simulink model "modelo_robot_6dof_dindir"  (R2023b)
settings: Solver=ode45  StartTime=0.0  StopTime=tsim  MaxStep=1e-2
undefined symbols (not defined in the file): robot_params, tau_L, tau_Rref
settings Model: Creator=HP  LastModifiedBy=HP

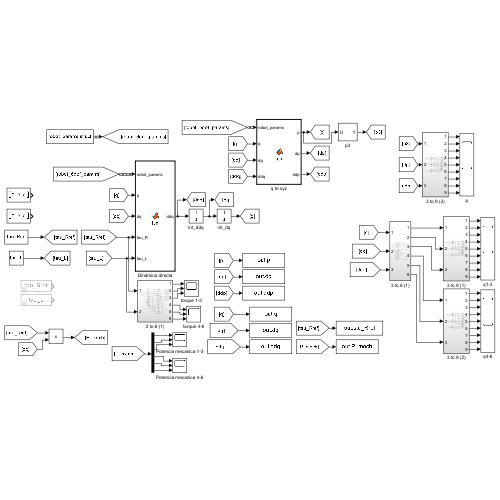
[thumbnail: Simulink's stored preview of the top-level diagram]
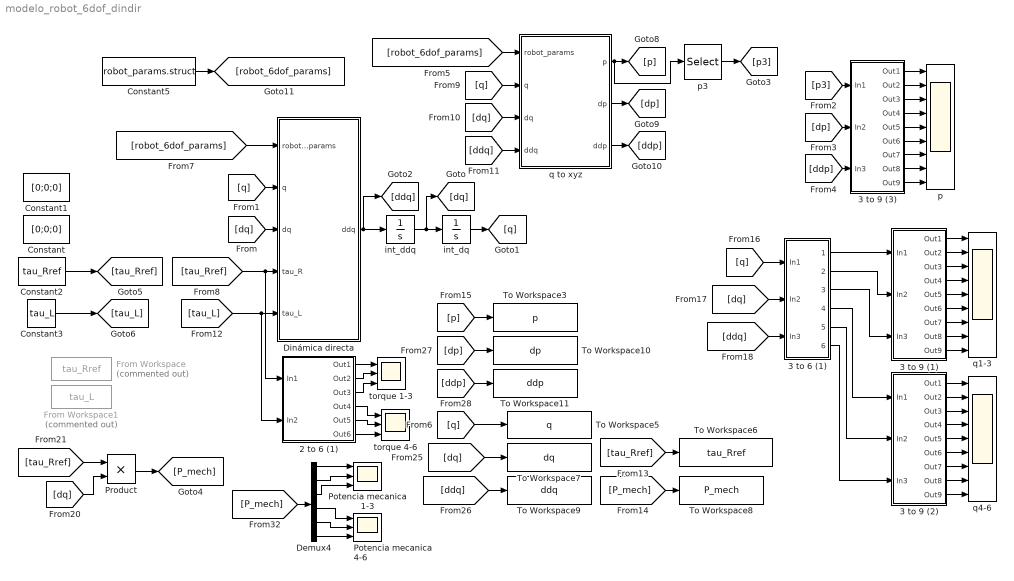
== system modelo_robot_6dof_dindir ==
  2 to 6 (1) : Subsystem
  3 to 6 (1) : Subsystem
  3 to 9 (1) : Subsystem
  3 to 9 (2) : Subsystem
  3 to 9 (3) : Subsystem
  Constant : Constant  Value=[0;0;0]
  Constant1 : Constant  Value=[0;0;0]
  Constant2 : Constant  Value=tau_Rref
  Constant3 : Constant  Value=tau_L
  Constant5 : Constant  Value=robot_params.struct  OutDataTypeStr=Bus: robot_params_bus
  Demux4 : Demux  Outputs=6
  Dinámica directa : MATLAB Function  TreatAsAtomicUnit=on
  From Workspace : FromWorkspace  Commented=on  VariableName=tau_Rref
  From Workspace1 : FromWorkspace  Commented=on  VariableName=tau_L
  Potencia mecanica 1-3 : Scope  NumInputPorts=3
  Potencia mecanica 4-6 : Scope  NumInputPorts=3
  Product : Product
  To Workspace10 : ToWorkspace  VariableName=dp  SaveFormat=Timeseries  SampleTime=-1
  To Workspace11 : ToWorkspace  VariableName=ddp  SaveFormat=Timeseries  SampleTime=-1
  To Workspace3 : ToWorkspace  VariableName=p  SaveFormat=Timeseries  SampleTime=-1
  To Workspace5 : ToWorkspace  VariableName=q  SaveFormat=Timeseries  SampleTime=-1
  To Workspace6 : ToWorkspace  VariableName=tau_Rref  SaveFormat=Timeseries  SampleTime=-1
  To Workspace7 : ToWorkspace  VariableName=dq  SaveFormat=Timeseries  SampleTime=-1
  To Workspace8 : ToWorkspace  VariableName=P_mech  SaveFormat=Timeseries  SampleTime=-1
  To Workspace9 : ToWorkspace  VariableName=ddq  SaveFormat=Timeseries  SampleTime=-1
  int_ddq : Integrator  InitialCondition=[0;0;0;0;0;0]
  int_dq : Integrator  InitialCondition=[0;-1.3744;0;1.669;0;0]
  p : Scope  NumInputPorts=9
  p3 : Selector  NumberOfDimensions=2  InputPortWidth=3  IndexOptions=Index vector (dialog),Index vector (dialog)  Indices=[1:3],3  OutputSizes=1,1
  q to xyz : MATLAB Function  TreatAsAtomicUnit=on
  q1-3 : Scope  NumInputPorts=9
  q4-6 : Scope  NumInputPorts=9
  torque 1-3 : Scope  NumInputPorts=3
  torque 4-6 : Scope  NumInputPorts=3
  wires:
  Dinámica directa/1(ddq) -> [ddq], int_ddq/1
  int_ddq/1 -> [dq], int_dq/1
  int_dq/1 -> [q]
  [dq] -> Dinámica directa/3(dq)
  [q] -> Dinámica directa/2(q)
  [tau_L] -> 2 to 6 (1)/2(In2), Dinámica directa/5(tau_L)
  Constant5/1 -> [robot_6dof_params]
  [robot_6dof_params] -> Dinámica directa/1(robot_params)
  [tau_Rref] -> 2 to 6 (1)/1(In1), Dinámica directa/4(tau_R)
  [ddq] -> q to xyz/4(ddq)
  q to xyz/1(p) -> p3/1, [p]
  q to xyz/3(ddp) -> [ddp]
  [dq] -> q to xyz/3(dq)
  [q] -> q to xyz/2(q)
  [robot_6dof_params] -> q to xyz/1(robot_params)
  q to xyz/2(dp) -> [dp]
  2 to 6 (1)/1(Out1) -> torque 1-3/1
  3 to 9 (3)/9(Out9) -> p/9
  3 to 9 (3)/7(Out7) -> p/7
  [dp] -> 3 to 9 (3)/2(In2)
  [ddp] -> 3 to 9 (3)/3(In3)
  3 to 9 (3)/8(Out8) -> p/8
  3 to 9 (3)/1(Out1) -> p/1
  3 to 9 (3)/5(Out5) -> p/5
  3 to 9 (3)/6(Out6) -> p/6
  3 to 9 (3)/4(Out4) -> p/4
  3 to 9 (3)/3(Out3) -> p/3
  3 to 9 (3)/2(Out2) -> p/2
  p3/1 -> [p3]
  [p3] -> 3 to 9 (3)/1(In1)
  2 to 6 (1)/2(Out2) -> torque 1-3/2
  2 to 6 (1)/3(Out3) -> torque 1-3/3
  Product/1 -> [P_mech]
  [dq] -> Product/2
  [tau_Rref] -> Product/1
  Constant2/1 -> [tau_Rref]
  Constant3/1 -> [tau_L]
  [ddq] -> To Workspace9/1
  [P_mech] -> To Workspace8/1
  [dq] -> To Workspace7/1
  [q] -> To Workspace5/1
  [tau_Rref] -> To Workspace6/1
  [dp] -> To Workspace10/1
  [ddp] -> To Workspace11/1
  [p] -> To Workspace3/1
  Demux4/3 -> Potencia mecanica 1-3/3
  Demux4/5 -> Potencia mecanica 4-6/2
  Demux4/2 -> Potencia mecanica 1-3/2
  [P_mech] -> Demux4/1
  Demux4/4 -> Potencia mecanica 4-6/1
  Demux4/1 -> Potencia mecanica 1-3/1
  Demux4/6 -> Potencia mecanica 4-6/3
  2 to 6 (1)/4(Out4) -> torque 4-6/1
  2 to 6 (1)/5(Out5) -> torque 4-6/2
  2 to 6 (1)/6(Out6) -> torque 4-6/3
  3 to 6 (1)/4(Out4) -> 3 to 9 (2)/1(In1)
  3 to 6 (1)/5(Out5) -> 3 to 9 (2)/2(In2)
  3 to 6 (1)/6(Out6) -> 3 to 9 (2)/3(In3)
  3 to 6 (1)/3(Out3) -> 3 to 9 (1)/3(In3)
  [ddq] -> 3 to 6 (1)/3(In3)
  [dq] -> 3 to 6 (1)/2(In2)
  3 to 6 (1)/2(Out2) -> 3 to 9 (1)/2(In2)
  [q] -> 3 to 6 (1)/1(In1)
  3 to 9 (2)/2(Out2) -> q4-6/2
  3 to 9 (2)/7(Out7) -> q4-6/7
  3 to 9 (2)/6(Out6) -> q4-6/6
  3 to 9 (2)/8(Out8) -> q4-6/8
  3 to 9 (2)/4(Out4) -> q4-6/4
  3 to 9 (2)/1(Out1) -> q4-6/1
  3 to 9 (1)/1(Out1) -> q1-3/1
  3 to 9 (2)/5(Out5) -> q4-6/5
  3 to 9 (1)/9(Out9) -> q1-3/9
  3 to 9 (1)/4(Out4) -> q1-3/4
  3 to 6 (1)/1(Out1) -> 3 to 9 (1)/1(In1)
  3 to 9 (1)/6(Out6) -> q1-3/6
  3 to 9 (2)/3(Out3) -> q4-6/3
  3 to 9 (1)/8(Out8) -> q1-3/8
  3 to 9 (1)/7(Out7) -> q1-3/7
  3 to 9 (1)/3(Out3) -> q1-3/3
  3 to 9 (1)/2(Out2) -> q1-3/2
  3 to 9 (2)/9(Out9) -> q4-6/9
  3 to 9 (1)/5(Out5) -> q1-3/5

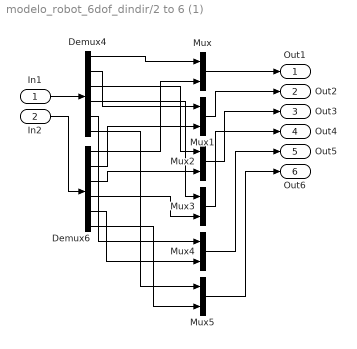
== system modelo_robot_6dof_dindir/2 to 6 (1) ==
  In1 : Inport
  In2 : Inport  Port=2
  Demux4 : Demux  Outputs=6
  Demux6 : Demux  Outputs=6
  Mux{,1..5} (6 alike) : Mux  Inputs=2
  Out1 : Outport
  Out2 : Outport  Port=2
  Out3 : Outport  Port=3
  Out4 : Outport  Port=4
  Out5 : Outport  Port=5
  Out6 : Outport  Port=6
  wires:
  In2/1 -> Demux6/1
  Demux4/3 -> Mux2/1
  Demux4/5 -> Mux4/1
  Demux4/6 -> Mux5/1
  Demux6/5 -> Mux4/2
  Demux4/1 -> Mux/1
  Demux6/6 -> Mux5/2
  In1/1 -> Demux4/1
  Demux4/4 -> Mux3/1
  Demux6/2 -> Mux1/2
  Demux6/4 -> Mux3/2
  Demux6/1 -> Mux/2
  Demux4/2 -> Mux1/1
  Demux6/3 -> Mux2/2
  Mux/1 -> Out1/1
  Mux1/1 -> Out2/1
  Mux2/1 -> Out3/1
  Mux3/1 -> Out4/1
  Mux4/1 -> Out5/1
  Mux5/1 -> Out6/1

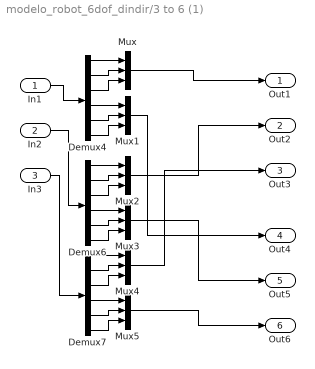
== system modelo_robot_6dof_dindir/3 to 6 (1) ==
  In1 : Inport
  In2 : Inport  Port=2
  In3 : Inport  Port=3
  Demux4 : Demux  Outputs=6
  Demux6 : Demux  Outputs=6
  Demux7 : Demux  Outputs=6
  Mux{,1..5} (6 alike) : Mux  Inputs=3
  Out1 : Outport
  Out2 : Outport  Port=2
  Out3 : Outport  Port=3
  Out4 : Outport  Port=4
  Out5 : Outport  Port=5
  Out6 : Outport  Port=6
  wires:
  Demux6/1 -> Mux2/1
  Demux6/3 -> Mux2/3
  Demux4/2 -> Mux/2
  Demux6/6 -> Mux3/3
  Demux6/2 -> Mux2/2
  Demux6/5 -> Mux3/2
  Mux/1 -> Out1/1
  In1/1 -> Demux4/1
  Demux6/4 -> Mux3/1
  Demux4/1 -> Mux/1
  Demux4/6 -> Mux1/3
  Demux4/4 -> Mux1/1
  Demux7/5 -> Mux5/2
  Demux4/3 -> Mux/3
  Demux4/5 -> Mux1/2
  Demux7/3 -> Mux4/3
  Demux7/1 -> Mux4/1
  Demux7/2 -> Mux4/2
  In3/1 -> Demux7/1
  Mux2/1 -> Out2/1
  Demux7/4 -> Mux5/1
  Demux7/6 -> Mux5/3
  In2/1 -> Demux6/1
  Mux5/1 -> Out6/1
  Mux1/1 -> Out4/1
  Mux4/1 -> Out3/1
  Mux3/1 -> Out5/1

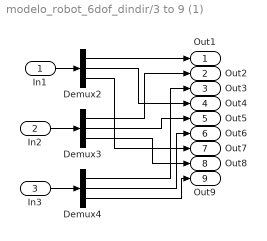
== system modelo_robot_6dof_dindir/3 to 9 (1) ==
  In1 : Inport
  In2 : Inport  Port=2
  In3 : Inport  Port=3
  Demux2 : Demux  Outputs=3
  Demux3 : Demux  Outputs=3
  Demux4 : Demux  Outputs=3
  Out1 : Outport
  Out2 : Outport  Port=2
  Out3 : Outport  Port=3
  Out4 : Outport  Port=4
  Out5 : Outport  Port=5
  Out6 : Outport  Port=6
  Out7 : Outport  Port=7
  Out8 : Outport  Port=8
  Out9 : Outport  Port=9
  wires:
  In3/1 -> Demux4/1
  Demux4/1 -> Out3/1
  Demux2/1 -> Out1/1
  Demux3/3 -> Out8/1
  Demux3/2 -> Out5/1
  Demux3/1 -> Out2/1
  In1/1 -> Demux2/1
  Demux2/3 -> Out7/1
  Demux4/3 -> Out9/1
  Demux4/2 -> Out6/1
  Demux2/2 -> Out4/1
  In2/1 -> Demux3/1

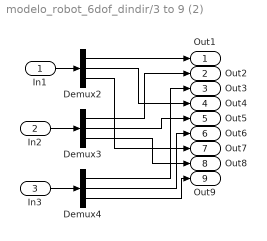
== system modelo_robot_6dof_dindir/3 to 9 (2) ==
  In1 : Inport
  In2 : Inport  Port=2
  In3 : Inport  Port=3
  Demux2 : Demux  Outputs=3
  Demux3 : Demux  Outputs=3
  Demux4 : Demux  Outputs=3
  Out1 : Outport
  Out2 : Outport  Port=2
  Out3 : Outport  Port=3
  Out4 : Outport  Port=4
  Out5 : Outport  Port=5
  Out6 : Outport  Port=6
  Out7 : Outport  Port=7
  Out8 : Outport  Port=8
  Out9 : Outport  Port=9
  wires:
  In3/1 -> Demux4/1
  Demux4/1 -> Out3/1
  Demux2/1 -> Out1/1
  Demux3/3 -> Out8/1
  Demux3/2 -> Out5/1
  Demux3/1 -> Out2/1
  In1/1 -> Demux2/1
  Demux2/3 -> Out7/1
  Demux4/3 -> Out9/1
  Demux4/2 -> Out6/1
  Demux2/2 -> Out4/1
  In2/1 -> Demux3/1

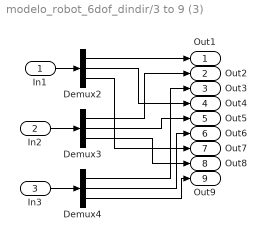
== system modelo_robot_6dof_dindir/3 to 9 (3) ==
  In1 : Inport
  In2 : Inport  Port=2
  In3 : Inport  Port=3
  Demux2 : Demux  Outputs=3
  Demux3 : Demux  Outputs=3
  Demux4 : Demux  Outputs=3
  Out1 : Outport
  Out2 : Outport  Port=2
  Out3 : Outport  Port=3
  Out4 : Outport  Port=4
  Out5 : Outport  Port=5
  Out6 : Outport  Port=6
  Out7 : Outport  Port=7
  Out8 : Outport  Port=8
  Out9 : Outport  Port=9
  wires:
  In3/1 -> Demux4/1
  Demux4/1 -> Out3/1
  Demux2/1 -> Out1/1
  Demux3/3 -> Out8/1
  Demux3/2 -> Out5/1
  Demux3/1 -> Out2/1
  In1/1 -> Demux2/1
  Demux2/3 -> Out7/1
  Demux4/3 -> Out9/1
  Demux4/2 -> Out6/1
  Demux2/2 -> Out4/1
  In2/1 -> Demux3/1

== matlab function modelo_robot_6dof_dindir/Dinámica directa ==
  data: robot_params input; q input size=[6,1]; ddq output size=[6,1]; dq input size=[6,1]; tau_R input size=[6,1]; tau_L input size=[6,1]
function ddq = fcn(robot_params,q,dq,tau_R,tau_L)

%l1 = robot_params.l(1);
l2 = robot_params.l(2);
l3 = robot_params.l(3);
%l4 = robot_params.l(4);
%l5 = robot_params.l(5);
%l6 = robot_params.l(6);

lc1 = robot_params.lc(1);
lc2 = robot_params.lc(2);
lc3 = robot_params.lc(3);
%lc4 = robot_params.lc(4);
%lc5 = robot_params.lc(5);
%lc6 = robot_params.lc(6);

d1 = robot_params.d(1);
d2 = robot_params.d(2);
d3 = robot_params.d(3);
d4 = robot_params.d(4);
d5 = robot_params.d(5);
d6 = robot_params.d(6);

%dc1 = robot_params.dc(1);
%dc2 = robot_params.dc(2);
%dc3 = robot_params.dc(3);
dc4 = robot_params.dc(4);
dc5 = robot_params.dc(5);
dc6 = robot_params.dc(6);

% yc1 = 0;%robot_params.yc(1);
% yc2 = 0;%robot_params.yc(2);
% yc3 = 0;%robot_params.yc(3);
% yc4 = 0;%robot_params.yc(4);
% yc5 = 0;%robot_params.yc(5);
% yc6 = 0;%robot_params.yc(6);

m1 = robot_params.m(1);
m2 = robot_params.m(2);
m3 = robot_params.m(3);
m4 = robot_params.m(4);
m5 = robot_params.m(5);
m6 = robot_params.m(6);

g = 9.81;

%Posiciones angulares
q1 = q(1);
q2 = q(2);
q3 = q(3);
q4 = q(4);
q5 = q(5);
q6 = q(6);

%Velocidades angulares
dq1 = dq(1);
dq2 = dq(2);
dq3 = dq(3);
dq4 = dq(4);
dq5 = dq(5);
dq6 = dq(6);

% Matriz de Inercia D: 

D = zeros(6,6);

D(1,1) = (d1*m1)/2 + (d2*m2)/2 + (d3*m3)/2 + (d4*m4)/2 + (d5*m5)/2 + (d6*m6)/2 + d4^2*m5 + d4^2*m6 + (d5^2*m6)/2 + dc4^2*m4 + (dc5^2*m5)/2 + (3*dc6^2*m6)/4 + (l2^2*m3)/2 + (l2^2*m4)/2 + (l2^2*m5)/2 + (l3^2*m4)/2 + (l2^2*m6)/2 + (l3^2*m5)/2 + (l3^2*m6)/2 + lc1^2*m1 + (lc2^2*m2)/2 + (lc3^2*m3)/2 - (dc6^2*m6*cos(2*q2 + 2*q3 + 2*q4 - 2*q5))/8 - (dc6^2*m6*cos(2*q2 + 2*q3 + 2*q4 + 2*q5))/8 - (d5^2*m6*cos(2*q2 + 2*q3 + 2*q4))/2 + (dc6^2*m6*cos(2*q5))/4 - (dc5^2*m5*cos(2*q2 + 2*q3 + 2*q4))/2 + (dc6^2*m6*cos(2*q2 + 2*q3 + 2*q4))/4 + (l2^2*m3*cos(2*q2))/2 + (l2^2*m4*cos(2*q2))/2 + (l2^2*m5*cos(2*q2))/2 + (l2^2*m6*cos(2*q2))/2 + (lc2^2*m2*cos(2*q2))/2 + (l3^2*m4*cos(2*q2 + 2*q3))/2 + (l3^2*m5*cos(2*q2 + 2*q3))/2 + (l3^2*m6*cos(2*q2 + 2*q3))/2 + (lc3^2*m3*cos(2*q2 + 2*q3))/2 + d5*l2*m6*sin(2*q2 + q3 + q4) + dc5*l2*m5*sin(2*q2 + q3 + q4) + (dc6*l2*m6*sin(q3 + q4 - q5))/2 + (d5*dc6*m6*cos(2*q2 + 2*q3 + 2*q4 + q5))/2 + d5*l2*m6*sin(q3 + q4) + dc5*l2*m5*sin(q3 + q4) - (dc6*l3*m6*sin(q4 + q5))/2 + (dc6*l3*m6*sin(2*q2 + 2*q3 + q4 - q5))/2 + 2*d4*dc6*m6*cos(q5) + l2*l3*m4*cos(q3) + l2*l3*m5*cos(q3) + l2*l3*m6*cos(q3) + l2*lc3*m3*cos(q3) + d5*l3*m6*sin(q4) + d5*l3*m6*sin(2*q2 + 2*q3 + q4) + dc5*l3*m5*sin(q4) + dc5*l3*m5*sin(2*q2 + 2*q3 + q4) - (dc6*l2*m6*sin(2*q2 + q3 + q4 + q5))/2 - (d5*dc6*m6*cos(2*q2 + 2*q3 + 2*q4 - q5))/2 + l2*l3*m4*cos(2*q2 + q3) + l2*l3*m5*cos(2*q2 + q3) + l2*l3*m6*cos(2*q2 + q3) + l2*lc3*m3*cos(2*q2 + q3) + (dc6*l3*m6*sin(q4 - q5))/2 - (dc6*l2*m6*sin(q3 + q4 + q5))/2 + (dc6*l2*m6*sin(2*q2 + q3 + q4 - q5))/2 - (dc6*l3*m6*sin(2*q2 + 2*q3 + q4 + q5))/2;
D(1,2) = (dc6^2*m6*cos(q2 + q3 + q4 - 2*q5))/4 - (dc6^2*m6*cos(q2 + q3 + q4 + 2*q5))/4 - (d4*dc6*m6*cos(q2 + q3 + q4 + q5))/2 + (d5*dc6*m6*cos(q2 + q3 + q4 + q5))/2 - (dc6*l3*m6*sin(q2 + q3 - q5))/2 - d4*l3*m5*sin(q2 + q3) - d4*l3*m6*sin(q2 + q3) - dc4*l3*m4*sin(q2 + q3) - (dc6*l2*m6*sin(q2 + q5))/2 + (d4*dc6*m6*cos(q2 + q3 + q4 - q5))/2 + (d5*dc6*m6*cos(q2 + q3 + q4 - q5))/2 - d4*l2*m5*sin(q2) - d4*l2*m6*sin(q2) - dc4*l2*m4*sin(q2) + d4*d5*m6*cos(q2 + q3 + q4) + d4*dc5*m5*cos(q2 + q3 + q4) - (dc6*l2*m6*sin(q2 - q5))/2 - (dc6*l3*m6*sin(q2 + q3 + q5))/2;
D(1,3) = (dc6^2*m6*cos(q2 + q3 + q4 - 2*q5))/4 - (dc6^2*m6*cos(q2 + q3 + q4 + 2*q5))/4 - (d4*dc6*m6*cos(q2 + q3 + q4 + q5))/2 + (d5*dc6*m6*cos(q2 + q3 + q4 + q5))/2 - (dc6*l3*m6*sin(q2 + q3 - q5))/2 - d4*l3*m5*sin(q2 + q3) - d4*l3*m6*sin(q2 + q3) - dc4*l3*m4*sin(q2 + q3) + (d4*dc6*m6*cos(q2 + q3 + q4 - q5))/2 + (d5*dc6*m6*cos(q2 + q3 + q4 - q5))/2 + d4*d5*m6*cos(q2 + q3 + q4) + d4*dc5*m5*cos(q2 + q3 + q4) - (dc6*l3*m6*sin(q2 + q3 + q5))/2;
D(1,4) = (dc6^2*m6*cos(q2 + q3 + q4 - 2*q5))/4 - (dc6^2*m6*cos(q2 + q3 + q4 + 2*q5))/4 - (d4*dc6*m6*cos(q2 + q3 + q4 + q5))/2 + (d5*dc6*m6*cos(q2 + q3 + q4 + q5))/2 + (d4*dc6*m6*cos(q2 + q3 + q4 - q5))/2 + (d5*dc6*m6*cos(q2 + q3 + q4 - q5))/2 + d4*d5*m6*cos(q2 + q3 + q4) + d4*dc5*m5*cos(q2 + q3 + q4);
D(1,5) = -(dc6*m6*(d4*cos(q2 + q3 + q4 + q5) + d5*cos(q2 + q3 + q4 + q5) + l3*sin(q2 + q3 - q5) - l2*sin(q2 + q5) + d4*cos(q2 + q3 + q4 - q5) - d5*cos(q2 + q3 + q4 - q5) + 2*dc6*cos(q2 + q3 + q4) + l2*sin(q2 - q5) - l3*sin(q2 + q3 + q5)))/2;
D(1,6) = 0;

D(2,1) = (dc6^2*m6*cos(q2 + q3 + q4 - 2*q5))/4 - (dc6^2*m6*cos(q2 + q3 + q4 + 2*q5))/4 - (d4*dc6*m6*cos(q2 + q3 + q4 + q5))/2 + (d5*dc6*m6*cos(q2 + q3 + q4 + q5))/2 - (dc6*l3*m6*sin(q2 + q3 - q5))/2 - d4*l3*m5*sin(q2 + q3) - d4*l3*m6*sin(q2 + q3) - dc4*l3*m4*sin(q2 + q3) - (dc6*l2*m6*sin(q2 + q5))/2 + (d4*dc6*m6*cos(q2 + q3 + q4 - q5))/2 + (d5*dc6*m6*cos(q2 + q3 + q4 - q5))/2 - d4*l2*m5*sin(q2) - d4*l2*m6*sin(q2) - dc4*l2*m4*sin(q2) + d4*d5*m6*cos(q2 + q3 + q4) + d4*dc5*m5*cos(q2 + q3 + q4) - (dc6*l2*m6*sin(q2 - q5))/2 - (dc6*l3*m6*sin(q2 + q3 + q5))/2;
D(2,2) = (d2*m2)/2 + (d3*m3)/2 + (d4*m4)/2 + (d5*m5)/2 + (d6*m6)/2 + d5^2*m6 + dc5^2*m5 + (dc6^2*m6)/2 + l2^2*m3 + l2^2*m4 + l2^2*m5 + l3^2*m4 + l2^2*m6 + l3^2*m5 + l3^2*m6 + lc2^2*m2 + lc3^2*m3 - (dc6^2*m6*cos(2*q5))/2 + 2*d5*l2*m6*sin(q3 + q4) + 2*dc5*l2*m5*sin(q3 + q4) + 2*l2*l3*m4*cos(q3) + 2*l2*l3*m5*cos(q3) + 2*l2*l3*m6*cos(q3) + 2*l2*lc3*m3*cos(q3) + 2*d5*l3*m6*sin(q4) + 2*dc5*l3*m5*sin(q4) - 2*dc6*l3*m6*cos(q4)*sin(q5) - 2*dc6*l2*m6*cos(q3)*cos(q4)*sin(q5) + 2*dc6*l2*m6*sin(q3)*sin(q4)*sin(q5);
D(2,3) = d5^2*m6 + dc5^2*m5 + (dc6^2*m6)/2 + l3^2*m4 + l3^2*m5 + l3^2*m6 + lc3^2*m3 - (dc6^2*m6*cos(2*q5))/2 + d5*l2*m6*sin(q3 + q4) + dc5*l2*m5*sin(q3 + q4) + l2*l3*m4*cos(q3) + l2*l3*m5*cos(q3) + l2*l3*m6*cos(q3) + l2*lc3*m3*cos(q3) + 2*d5*l3*m6*sin(q4) + 2*dc5*l3*m5*sin(q4) - 2*dc6*l3*m6*cos(q4)*sin(q5) - dc6*l2*m6*cos(q3)*cos(q4)*sin(q5) + dc6*l2*m6*sin(q3)*sin(q4)*sin(q5);
D(2,4) = d5^2*m6 + dc5^2*m5 + (dc6^2*m6)/2 - (dc6^2*m6*cos(2*q5))/2 + d5*l2*m6*sin(q3 + q4) + dc5*l2*m5*sin(q3 + q4) + d5*l3*m6*sin(q4) + dc5*l3*m5*sin(q4) - dc6*l3*m6*cos(q4)*sin(q5) - dc6*l2*m6*cos(q3)*cos(q4)*sin(q5) + dc6*l2*m6*sin(q3)*sin(q4)*sin(q5);
D(2,5) = -dc6*m6*cos(q5)*(d5 + l2*sin(q3 + q4) + l3*sin(q4));
D(2,6) = 0;

D(3,1) = (dc6^2*m6*cos(q2 + q3 + q4 - 2*q5))/4 - (dc6^2*m6*cos(q2 + q3 + q4 + 2*q5))/4 - (d4*dc6*m6*cos(q2 + q3 + q4 + q5))/2 + (d5*dc6*m6*cos(q2 + q3 + q4 + q5))/2 - (dc6*l3*m6*sin(q2 + q3 - q5))/2 - d4*l3*m5*sin(q2 + q3) - d4*l3*m6*sin(q2 + q3) - dc4*l3*m4*sin(q2 + q3) + (d4*dc6*m6*cos(q2 + q3 + q4 - q5))/2 + (d5*dc6*m6*cos(q2 + q3 + q4 - q5))/2 + d4*d5*m6*cos(q2 + q3 + q4) + d4*dc5*m5*cos(q2 + q3 + q4) - (dc6*l3*m6*sin(q2 + q3 + q5))/2;
D(3,2) = d5^2*m6 + dc5^2*m5 + (dc6^2*m6)/2 + l3^2*m4 + l3^2*m5 + l3^2*m6 + lc3^2*m3 - (dc6^2*m6*cos(2*q5))/2 + d5*l2*m6*sin(q3 + q4) + dc5*l2*m5*sin(q3 + q4) + l2*l3*m4*cos(q3) + l2*l3*m5*cos(q3) + l2*l3*m6*cos(q3) + l2*lc3*m3*cos(q3) + 2*d5*l3*m6*sin(q4) + 2*dc5*l3*m5*sin(q4) - 2*dc6*l3*m6*cos(q4)*sin(q5) - dc6*l2*m6*cos(q3)*cos(q4)*sin(q5) + dc6*l2*m6*sin(q3)*sin(q4)*sin(q5);
D(3,3) = (d3*m3)/2 + (d4*m4)/2 + (d5*m5)/2 + (d6*m6)/2 + d5^2*m6 + dc5^2*m5 + l3^2*m4 + l3^2*m5 + l3^2*m6 + lc3^2*m3 + dc6^2*m6*sin(q5)^2 + 2*d5*l3*m6*sin(q4) + 2*dc5*l3*m5*sin(q4) - 2*dc6*l3*m6*cos(q4)*sin(q5);
D(3,4) = d5^2*m6 + dc5^2*m5 + dc6^2*m6*sin(q5)^2 + d5*l3*m6*sin(q4) + dc5*l3*m5*sin(q4) - dc6*l3*m6*cos(q4)*sin(q5);
D(3,5) = -dc6*m6*cos(q5)*(d5 + l3*sin(q4));
D(3,6) = 0;

D(4,1) = (dc6^2*m6*cos(q2 + q3 + q4 - 2*q5))/4 - (dc6^2*m6*cos(q2 + q3 + q4 + 2*q5))/4 - (d4*dc6*m6*cos(q2 + q3 + q4 + q5))/2 + (d5*dc6*m6*cos(q2 + q3 + q4 + q5))/2 + (d4*dc6*m6*cos(q2 + q3 + q4 - q5))/2 + (d5*dc6*m6*cos(q2 + q3 + q4 - q5))/2 + d4*d5*m6*cos(q2 + q3 + q4) + d4*dc5*m5*cos(q2 + q3 + q4);
D(4,2) = d5^2*m6 + dc5^2*m5 + (dc6^2*m6)/2 - (dc6^2*m6*cos(2*q5))/2 + d5*l2*m6*sin(q3 + q4) + dc5*l2*m5*sin(q3 + q4) + d5*l3*m6*sin(q4) + dc5*l3*m5*sin(q4) - dc6*l3*m6*cos(q4)*sin(q5) - dc6*l2*m6*cos(q3)*cos(q4)*sin(q5) + dc6*l2*m6*sin(q3)*sin(q4)*sin(q5);
D(4,3) = d5^2*m6 + dc5^2*m5 + dc6^2*m6*sin(q5)^2 + d5*l3*m6*sin(q4) + dc5*l3*m5*sin(q4) - dc6*l3*m6*cos(q4)*sin(q5);
D(4,4) = (d4*m4)/2 + (d5*m5)/2 + (d6*m6)/2 + d5^2*m6 + dc5^2*m5 + dc6^2*m6 - dc6^2*m6*cos(q5)^2;
D(4,5) = -d5*dc6*m6*cos(q5);
D(4,6) = 0;

D(5,1) = -(dc6*m6*(d4*cos(q2 + q3 + q4 + q5) + d5*cos(q2 + q3 + q4 + q5) + l3*sin(q2 + q3 - q5) - l2*sin(q2 + q5) + d4*cos(q2 + q3 + q4 - q5) - d5*cos(q2 + q3 + q4 - q5) + 2*dc6*cos(q2 + q3 + q4) + l2*sin(q2 - q5) - l3*sin(q2 + q3 + q5)))/2;
D(5,2) = -dc6*m6*cos(q5)*(d5 + l2*sin(q3 + q4) + l3*sin(q4));
D(5,3) = -dc6*m6*cos(q5)*(d5 + l3*sin(q4));
D(5,4) = -d5*dc6*m6*cos(q5);
D(5,5) = (d5*m5)/2 + (d6*m6)/2 + dc6^2*m6;
D(5,6) = 0;

D(6,1) = 0;
D(6,2) = 0;
D(6,3) = 0;
D(6,4) = 0;
D(6,5) = 0;
D(6,6) = 1;


% Matriz de Coriollis C: 

C = zeros(6,6);

C(1,1) = 0;
C(1,2) = (dc6^2*dq1*m6*sin(2*q2 + 2*q3 + 2*q4 - 2*q5))/4 + (dc6^2*dq1*m6*sin(2*q2 + 2*q3 + 2*q4 + 2*q5))/4 + d5^2*dq1*m6*sin(2*q2 + 2*q3 + 2*q4) + dc5^2*dq1*m5*sin(2*q2 + 2*q3 + 2*q4) - (dc6^2*dq1*m6*sin(2*q2 + 2*q3 + 2*q4))/2 - dq1*l2^2*m3*sin(2*q2) - dq1*l2^2*m4*sin(2*q2) - dq1*l2^2*m5*sin(2*q2) - dq1*l2^2*m6*sin(2*q2) - dq1*lc2^2*m2*sin(2*q2) - dq1*l3^2*m4*sin(2*q2 + 2*q3) - dq1*l3^2*m5*sin(2*q2 + 2*q3) - dq1*l3^2*m6*sin(2*q2 + 2*q3) - dq1*lc3^2*m3*sin(2*q2 + 2*q3) - (dc6^2*dq2*m6*sin(q2 + q3 + q4 - 2*q5))/4 + (dc6^2*dq2*m6*sin(q2 + q3 + q4 + 2*q5))/4 - (dc6*dq2*l2*m6*cos(q2 - q5))/2 + d5*dc6*dq1*m6*sin(2*q2 + 2*q3 + 2*q4 - q5) - (dc6*dq2*l3*m6*cos(q2 + q3 + q5))/2 - 2*dq1*l2*l3*m4*sin(2*q2 + q3) - 2*dq1*l2*l3*m5*sin(2*q2 + q3) - 2*dq1*l2*l3*m6*sin(2*q2 + q3) - 2*dq1*l2*lc3*m3*sin(2*q2 + q3) - d4*d5*dq2*m6*sin(q2 + q3 + q4) - d4*dc5*dq2*m5*sin(q2 + q3 + q4) + dc6*dq1*l2*m6*cos(2*q2 + q3 + q4 - q5) - dc6*dq1*l3*m6*cos(2*q2 + 2*q3 + q4 + q5) + 2*d5*dq1*l2*m6*cos(2*q2 + q3 + q4) + 2*dc5*dq1*l2*m5*cos(2*q2 + q3 + q4) - (dc6*dq2*l3*m6*cos(q2 + q3 - q5))/2 + (d4*dc6*dq2*m6*sin(q2 + q3 + q4 + q5))/2 - (d5*dc6*dq2*m6*sin(q2 + q3 + q4 + q5))/2 - d4*dq2*l3*m5*cos(q2 + q3) - d4*dq2*l3*m6*cos(q2 + q3) - dc4*dq2*l3*m4*cos(q2 + q3) - (dc6*dq2*l2*m6*cos(q2 + q5))/2 + dc6*dq1*l3*m6*cos(2*q2 + 2*q3 + q4 - q5) - d5*dc6*dq1*m6*sin(2*q2 + 2*q3 + 2*q4 + q5) - d4*dq2*l2*m5*cos(q2) - d4*dq2*l2*m6*cos(q2) + 2*d5*dq1*l3*m6*cos(2*q2 + 2*q3 + q4) - dc4*dq2*l2*m4*cos(q2) + 2*dc5*dq1*l3*m5*cos(2*q2 + 2*q3 + q4) - dc6*dq1*l2*m6*cos(2*q2 + q3 + q4 + q5) - (d4*dc6*dq2*m6*sin(q2 + q3 + q4 - q5))/2 - (d5*dc6*dq2*m6*sin(q2 + q3 + q4 - q5))/2;
C(1,3) = (dc6^2*dq1*m6*sin(2*q2 + 2*q3 + 2*q4 - 2*q5))/4 + (dc6^2*dq1*m6*sin(2*q2 + 2*q3 + 2*q4 + 2*q5))/4 + d5^2*dq1*m6*sin(2*q2 + 2*q3 + 2*q4) + dc5^2*dq1*m5*sin(2*q2 + 2*q3 + 2*q4) - (dc6^2*dq1*m6*sin(2*q2 + 2*q3 + 2*q4))/2 - dq1*l3^2*m4*sin(2*q2 + 2*q3) - dq1*l3^2*m5*sin(2*q2 + 2*q3) - dq1*l3^2*m6*sin(2*q2 + 2*q3) - dq1*lc3^2*m3*sin(2*q2 + 2*q3) - (dc6^2*dq2*m6*sin(q2 + q3 + q4 - 2*q5))/2 + (dc6^2*dq2*m6*sin(q2 + q3 + q4 + 2*q5))/2 - (dc6^2*dq3*m6*sin(q2 + q3 + q4 - 2*q5))/4 + (dc6^2*dq3*m6*sin(q2 + q3 + q4 + 2*q5))/4 + d5*dc6*dq1*m6*sin(2*q2 + 2*q3 + 2*q4 - q5) - (dc6*dq1*l2*m6*cos(q3 + q4 + q5))/2 - dc6*dq2*l3*m6*cos(q2 + q3 + q5) - (dc6*dq3*l3*m6*cos(q2 + q3 + q5))/2 - dq1*l2*l3*m4*sin(2*q2 + q3) - dq1*l2*l3*m5*sin(2*q2 + q3) - dq1*l2*l3*m6*sin(2*q2 + q3) - dq1*l2*lc3*m3*sin(2*q2 + q3) - 2*d4*d5*dq2*m6*sin(q2 + q3 + q4) - d4*d5*dq3*m6*sin(q2 + q3 + q4) - 2*d4*dc5*dq2*m5*sin(q2 + q3 + q4) - d4*dc5*dq3*m5*sin(q2 + q3 + q4) + (dc6*dq1*l2*m6*cos(2*q2 + q3 + q4 - q5))/2 - dc6*dq1*l3*m6*cos(2*q2 + 2*q3 + q4 + q5) + d5*dq1*l2*m6*cos(2*q2 + q3 + q4) + dc5*dq1*l2*m5*cos(2*q2 + q3 + q4) + (dc6*dq1*l2*m6*cos(q3 + q4 - q5))/2 - dc6*dq2*l3*m6*cos(q2 + q3 - q5) - (dc6*dq3*l3*m6*cos(q2 + q3 - q5))/2 + d4*dc6*dq2*m6*sin(q2 + q3 + q4 + q5) + (d4*dc6*dq3*m6*sin(q2 + q3 + q4 + q5))/2 - d5*dc6*dq2*m6*sin(q2 + q3 + q4 + q5) - (d5*dc6*dq3*m6*sin(q2 + q3 + q4 + q5))/2 - 2*d4*dq2*l3*m5*cos(q2 + q3) - 2*d4*dq2*l3*m6*cos(q2 + q3) - d4*dq3*l3*m5*cos(q2 + q3) - d4*dq3*l3*m6*cos(q2 + q3) + d5*dq1*l2*m6*cos(q3 + q4) - 2*dc4*dq2*l3*m4*cos(q2 + q3) - dc4*dq3*l3*m4*cos(q2 + q3) + dc5*dq1*l2*m5*cos(q3 + q4) + dc6*dq1*l3*m6*cos(2*q2 + 2*q3 + q4 - q5) - d5*dc6*dq1*m6*sin(2*q2 + 2*q3 + 2*q4 + q5) + 2*d5*dq1*l3*m6*cos(2*q2 + 2*q3 + q4) + 2*dc5*dq1*l3*m5*cos(2*q2 + 2*q3 + q4) - (dc6*dq1*l2*m6*cos(2*q2 + q3 + q4 + q5))/2 - dq1*l2*l3*m4*sin(q3) - dq1*l2*l3*m5*sin(q3) - dq1*l2*l3*m6*sin(q3) - dq1*l2*lc3*m3*sin(q3) - d4*dc6*dq2*m6*sin(q2 + q3 + q4 - q5) - (d4*dc6*dq3*m6*sin(q2 + q3 + q4 - q5))/2 - d5*dc6*dq2*m6*sin(q2 + q3 + q4 - q5) - (d5*dc6*dq3*m6*sin(q2 + q3 + q4 - q5))/2;
C(1,4) = (dc6^2*dq1*m6*sin(2*q2 + 2*q3 + 2*q4 - 2*q5))/4 + (dc6^2*dq1*m6*sin(2*q2 + 2*q3 + 2*q4 + 2*q5))/4 + d5^2*dq1*m6*sin(2*q2 + 2*q3 + 2*q4) + dc5^2*dq1*m5*sin(2*q2 + 2*q3 + 2*q4) - (dc6^2*dq1*m6*sin(2*q2 + 2*q3 + 2*q4))/2 - (dc6^2*dq2*m6*sin(q2 + q3 + q4 - 2*q5))/2 + (dc6^2*dq2*m6*sin(q2 + q3 + q4 + 2*q5))/2 - (dc6^2*dq3*m6*sin(q2 + q3 + q4 - 2*q5))/2 + (dc6^2*dq3*m6*sin(q2 + q3 + q4 + 2*q5))/2 - (dc6^2*dq4*m6*sin(q2 + q3 + q4 - 2*q5))/4 + (dc6^2*dq4*m6*sin(q2 + q3 + q4 + 2*q5))/4 + (dc6*dq1*l3*m6*cos(q4 - q5))/2 + d5*dc6*dq1*m6*sin(2*q2 + 2*q3 + 2*q4 - q5) - (dc6*dq1*l2*m6*cos(q3 + q4 + q5))/2 - 2*d4*d5*dq2*m6*sin(q2 + q3 + q4) - 2*d4*d5*dq3*m6*sin(q2 + q3 + q4) - d4*d5*dq4*m6*sin(q2 + q3 + q4) - 2*d4*dc5*dq2*m5*sin(q2 + q3 + q4) - 2*d4*dc5*dq3*m5*sin(q2 + q3 + q4) - d4*dc5*dq4*m5*sin(q2 + q3 + q4) + (dc6*dq1*l2*m6*cos(2*q2 + q3 + q4 - q5))/2 - (dc6*dq1*l3*m6*cos(2*q2 + 2*q3 + q4 + q5))/2 + d5*dq1*l2*m6*cos(2*q2 + q3 + q4) + dc5*dq1*l2*m5*cos(2*q2 + q3 + q4) + (dc6*dq1*l2*m6*cos(q3 + q4 - q5))/2 + d4*dc6*dq2*m6*sin(q2 + q3 + q4 + q5) + d4*dc6*dq3*m6*sin(q2 + q3 + q4 + q5) - d5*dc6*dq2*m6*sin(q2 + q3 + q4 + q5) + (d4*dc6*dq4*m6*sin(q2 + q3 + q4 + q5))/2 - d5*dc6*dq3*m6*sin(q2 + q3 + q4 + q5) - (d5*dc6*dq4*m6*sin(q2 + q3 + q4 + q5))/2 + d5*dq1*l2*m6*cos(q3 + q4) + dc5*dq1*l2*m5*cos(q3 + q4) - (dc6*dq1*l3*m6*cos(q4 + q5))/2 + (dc6*dq1*l3*m6*cos(2*q2 + 2*q3 + q4 - q5))/2 - d5*dc6*dq1*m6*sin(2*q2 + 2*q3 + 2*q4 + q5) + d5*dq1*l3*m6*cos(q4) + d5*dq1*l3*m6*cos(2*q2 + 2*q3 + q4) + dc5*dq1*l3*m5*cos(q4) + dc5*dq1*l3*m5*cos(2*q2 + 2*q3 + q4) - (dc6*dq1*l2*m6*cos(2*q2 + q3 + q4 + q5))/2 - d4*dc6*dq2*m6*sin(q2 + q3 + q4 - q5) - d4*dc6*dq3*m6*sin(q2 + q3 + q4 - q5) - d5*dc6*dq2*m6*sin(q2 + q3 + q4 - q5) - (d4*dc6*dq4*m6*sin(q2 + q3 + q4 - q5))/2 - d5*dc6*dq3*m6*sin(q2 + q3 + q4 - q5) - (d5*dc6*dq4*m6*sin(q2 + q3 + q4 - q5))/2;
C(1,5) = (dc6*m6*(4*d4*dq2*sin(q2 + q3 + q4 - q5) - 2*dq1*l2*cos(2*q2 + q3 + q4 + q5) - 8*d4*dq1*sin(q5) + 4*d4*dq3*sin(q2 + q3 + q4 - q5) + 4*d4*dq4*sin(q2 + q3 + q4 - q5) - 2*d4*dq5*sin(q2 + q3 + q4 - q5) + 2*d5*dq5*sin(q2 + q3 + q4 - q5) + 2*dc6*dq2*sin(q2 + q3 + q4 - 2*q5) + 2*dc6*dq2*sin(q2 + q3 + q4 + 2*q5) + 2*dc6*dq3*sin(q2 + q3 + q4 - 2*q5) + 2*dc6*dq3*sin(q2 + q3 + q4 + 2*q5) + 2*dc6*dq4*sin(q2 + q3 + q4 - 2*q5) + 2*dc6*dq4*sin(q2 + q3 + q4 + 2*q5) - 2*dq1*l3*cos(q4 - q5) + 2*dq5*l2*cos(q2 - q5) - 2*d5*dq1*sin(2*q2 + 2*q3 + 2*q4 - q5) - dc6*dq1*sin(2*q2 + 2*q3 + 2*q4 - 2*q5) + dc6*dq1*sin(2*q2 + 2*q3 + 2*q4 + 2*q5) - 2*dq1*l2*cos(q3 + q4 + q5) + 2*dq5*l3*cos(q2 + q3 + q5) + 4*dc6*dq2*sin(q2 + q3 + q4) + 4*dc6*dq3*sin(q2 + q3 + q4) + 4*dc6*dq4*sin(q2 + q3 + q4) - 2*dc6*dq1*sin(2*q5) - 2*dq1*l2*cos(2*q2 + q3 + q4 - q5) - 2*dq1*l3*cos(2*q2 + 2*q3 + q4 + q5) - 2*dq1*l2*cos(q3 + q4 - q5) + 2*dq5*l3*cos(q2 + q3 - q5) + 4*d4*dq2*sin(q2 + q3 + q4 + q5) + 4*d4*dq3*sin(q2 + q3 + q4 + q5) + 4*d4*dq4*sin(q2 + q3 + q4 + q5) + 2*d4*dq5*sin(q2 + q3 + q4 + q5) + 2*d5*dq5*sin(q2 + q3 + q4 + q5) - 2*dq1*l3*cos(q4 + q5) + 2*dq5*l2*cos(q2 + q5) - 2*dq1*l3*cos(2*q2 + 2*q3 + q4 - q5) - 2*d5*dq1*sin(2*q2 + 2*q3 + 2*q4 + q5)))/4;
C(1,6) = 0;

C(2,1) = (dc6^2*dq1*m6*sin(2*q2 + 2*q3 + 2*q4))/4 - (dc6^2*dq1*m6*sin(2*q2 + 2*q3 + 2*q4 + 2*q5))/8 - (d5^2*dq1*m6*sin(2*q2 + 2*q3 + 2*q4))/2 - (dc5^2*dq1*m5*sin(2*q2 + 2*q3 + 2*q4))/2 - (dc6^2*dq1*m6*sin(2*q2 + 2*q3 + 2*q4 - 2*q5))/8 + (dq1*l2^2*m3*sin(2*q2))/2 + (dq1*l2^2*m4*sin(2*q2))/2 + (dq1*l2^2*m5*sin(2*q2))/2 + (dq1*l2^2*m6*sin(2*q2))/2 + (dq1*lc2^2*m2*sin(2*q2))/2 + (dq1*l3^2*m4*sin(2*q2 + 2*q3))/2 + (dq1*l3^2*m5*sin(2*q2 + 2*q3))/2 + (dq1*l3^2*m6*sin(2*q2 + 2*q3))/2 + (dq1*lc3^2*m3*sin(2*q2 + 2*q3))/2 - (d5*dc6*dq1*m6*sin(2*q2 + 2*q3 + 2*q4 - q5))/2 + dq1*l2*l3*m4*sin(2*q2 + q3) + dq1*l2*l3*m5*sin(2*q2 + q3) + dq1*l2*l3*m6*sin(2*q2 + q3) + dq1*l2*lc3*m3*sin(2*q2 + q3) - (dc6*dq1*l2*m6*cos(2*q2 + q3 + q4 - q5))/2 + (dc6*dq1*l3*m6*cos(2*q2 + 2*q3 + q4 + q5))/2 - d5*dq1*l2*m6*cos(2*q2 + q3 + q4) - dc5*dq1*l2*m5*cos(2*q2 + q3 + q4) - (dc6*dq1*l3*m6*cos(2*q2 + 2*q3 + q4 - q5))/2 + (d5*dc6*dq1*m6*sin(2*q2 + 2*q3 + 2*q4 + q5))/2 - d5*dq1*l3*m6*cos(2*q2 + 2*q3 + q4) - dc5*dq1*l3*m5*cos(2*q2 + 2*q3 + q4) + (dc6*dq1*l2*m6*cos(2*q2 + q3 + q4 + q5))/2;
C(2,2) = 0;
C(2,3) = -l2*(2*dq2 + dq3)*(l3*m4*sin(q3) + l3*m5*sin(q3) + l3*m6*sin(q3) + lc3*m3*sin(q3) - d5*m6*cos(q3 + q4) - dc5*m5*cos(q3 + q4) - dc6*m6*cos(q3)*sin(q4)*sin(q5) - dc6*m6*cos(q4)*sin(q3)*sin(q5));
C(2,4) = (dc6*dq4*l3*m6*cos(q4 - q5))/2 + 2*d5*dq2*l2*m6*cos(q3 + q4) + 2*d5*dq3*l2*m6*cos(q3 + q4) + d5*dq4*l2*m6*cos(q3 + q4) + 2*dc5*dq2*l2*m5*cos(q3 + q4) + 2*dc5*dq3*l2*m5*cos(q3 + q4) + dc5*dq4*l2*m5*cos(q3 + q4) - (dc6*dq4*l3*m6*cos(q4 + q5))/2 + 2*d5*dq2*l3*m6*cos(q4) + 2*d5*dq3*l3*m6*cos(q4) + d5*dq4*l3*m6*cos(q4) + 2*dc5*dq2*l3*m5*cos(q4) + 2*dc5*dq3*l3*m5*cos(q4) + dc5*dq4*l3*m5*cos(q4) + 2*dc6*dq2*l3*m6*sin(q4)*sin(q5) + 2*dc6*dq3*l3*m6*sin(q4)*sin(q5) + 2*dc6*dq2*l2*m6*cos(q3)*sin(q4)*sin(q5) + 2*dc6*dq2*l2*m6*cos(q4)*sin(q3)*sin(q5) + 2*dc6*dq3*l2*m6*cos(q3)*sin(q4)*sin(q5) + 2*dc6*dq3*l2*m6*cos(q4)*sin(q3)*sin(q5) + dc6*dq4*l2*m6*cos(q3)*sin(q4)*sin(q5) + dc6*dq4*l2*m6*cos(q4)*sin(q3)*sin(q5);
C(2,5) = -(dc6*m6*(2*dq2*l3*cos(q4 - q5) - 2*d5*dq1*sin(q2 + q3 + q4 - q5) - dc6*dq1*sin(q2 + q3 + q4 - 2*q5) - dc6*dq1*sin(q2 + q3 + q4 + 2*q5) - 2*dq1*l2*cos(q2 - q5) - 2*d5*dq5*sin(q5) + 2*dq3*l3*cos(q4 - q5) + 2*dq4*l3*cos(q4 - q5) - dq5*l3*cos(q4 - q5) + 2*dq1*l3*cos(q2 + q3 + q5) + 2*dq2*l2*cos(q3 + q4 + q5) + 2*dq3*l2*cos(q3 + q4 + q5) + 2*dq4*l2*cos(q3 + q4 + q5) + dq5*l2*cos(q3 + q4 + q5) + 2*dc6*dq1*sin(q2 + q3 + q4) - 2*dc6*dq2*sin(2*q5) - 2*dc6*dq3*sin(2*q5) - 2*dc6*dq4*sin(2*q5) - 2*dq1*l3*cos(q2 + q3 - q5) + 2*dq2*l2*cos(q3 + q4 - q5) + 2*dq3*l2*cos(q3 + q4 - q5) + 2*dq4*l2*cos(q3 + q4 - q5) - dq5*l2*cos(q3 + q4 - q5) + 2*d5*dq1*sin(q2 + q3 + q4 + q5) + 2*dq1*l2*cos(q2 + q5) + 2*dq2*l3*cos(q4 + q5) + 2*dq3*l3*cos(q4 + q5) + 2*dq4*l3*cos(q4 + q5) + dq5*l3*cos(q4 + q5)))/2;
C(2,6) = 0;

C(3,1) = (dc6^2*dq1*m6*sin(2*q2 + 2*q3 + 2*q4))/4 - (dc6^2*dq1*m6*sin(2*q2 + 2*q3 + 2*q4 + 2*q5))/8 - (d5^2*dq1*m6*sin(2*q2 + 2*q3 + 2*q4))/2 - (dc5^2*dq1*m5*sin(2*q2 + 2*q3 + 2*q4))/2 - (dc6^2*dq1*m6*sin(2*q2 + 2*q3 + 2*q4 - 2*q5))/8 + (dq1*l3^2*m4*sin(2*q2 + 2*q3))/2 + (dq1*l3^2*m5*sin(2*q2 + 2*q3))/2 + (dq1*l3^2*m6*sin(2*q2 + 2*q3))/2 + (dq1*lc3^2*m3*sin(2*q2 + 2*q3))/2 - (d5*dc6*dq1*m6*sin(2*q2 + 2*q3 + 2*q4 - q5))/2 + (dc6*dq1*l2*m6*cos(q3 + q4 + q5))/4 + (dq1*l2*l3*m4*sin(2*q2 + q3))/2 + (dq1*l2*l3*m5*sin(2*q2 + q3))/2 + (dq1*l2*l3*m6*sin(2*q2 + q3))/2 + (dq1*l2*lc3*m3*sin(2*q2 + q3))/2 - (dc6*dq1*l2*m6*cos(2*q2 + q3 + q4 - q5))/4 + (dc6*dq1*l3*m6*cos(2*q2 + 2*q3 + q4 + q5))/2 - (d5*dq1*l2*m6*cos(2*q2 + q3 + q4))/2 - (dc5*dq1*l2*m5*cos(2*q2 + q3 + q4))/2 - (dc6*dq1*l2*m6*cos(q3 + q4 - q5))/4 - (d5*dq1*l2*m6*cos(q3 + q4))/2 - (dc5*dq1*l2*m5*cos(q3 + q4))/2 - (dc6*dq1*l3*m6*cos(2*q2 + 2*q3 + q4 - q5))/2 + (d5*dc6*dq1*m6*sin(2*q2 + 2*q3 + 2*q4 + q5))/2 - d5*dq1*l3*m6*cos(2*q2 + 2*q3 + q4) - dc5*dq1*l3*m5*cos(2*q2 + 2*q3 + q4) + (dc6*dq1*l2*m6*cos(2*q2 + q3 + q4 + q5))/4 + (dq1*l2*l3*m4*sin(q3))/2 + (dq1*l2*l3*m5*sin(q3))/2 + (dq1*l2*l3*m6*sin(q3))/2 + (dq1*l2*lc3*m3*sin(q3))/2;
C(3,2) = dq2*l2*(l3*m4*sin(q3) + l3*m5*sin(q3) + l3*m6*sin(q3) + lc3*m3*sin(q3) - d5*m6*cos(q3 + q4) - dc5*m5*cos(q3 + q4) - dc6*m6*cos(q3)*sin(q4)*sin(q5) - dc6*m6*cos(q4)*sin(q3)*sin(q5));
C(3,3) = 0;
C(3,4) = l3*(2*dq2 + 2*dq3 + dq4)*(d5*m6*cos(q4) + dc5*m5*cos(q4) + dc6*m6*sin(q4)*sin(q5));
C(3,5) = -dc6*m6*(dq2*l3*cos(q4 - q5) - d5*dq1*sin(q2 + q3 + q4 - q5) - (dc6*dq1*sin(q2 + q3 + q4 - 2*q5))/2 - (dc6*dq1*sin(q2 + q3 + q4 + 2*q5))/2 - d5*dq5*sin(q5) + dq3*l3*cos(q4 - q5) + dq4*l3*cos(q4 - q5) - (dq5*l3*cos(q4 - q5))/2 + dq1*l3*cos(q2 + q3 + q5) + dc6*dq1*sin(q2 + q3 + q4) - dc6*dq2*sin(2*q5) - dc6*dq3*sin(2*q5) - dc6*dq4*sin(2*q5) - dq1*l3*cos(q2 + q3 - q5) + d5*dq1*sin(q2 + q3 + q4 + q5) + dq2*l3*cos(q4 + q5) + dq3*l3*cos(q4 + q5) + dq4*l3*cos(q4 + q5) + (dq5*l3*cos(q4 + q5))/2);
C(3,6) = 0;

C(4,1) = (dc6^2*dq1*m6*sin(2*q2 + 2*q3 + 2*q4))/4 - (dc6^2*dq1*m6*sin(2*q2 + 2*q3 + 2*q4 + 2*q5))/8 - (d5^2*dq1*m6*sin(2*q2 + 2*q3 + 2*q4))/2 - (dc5^2*dq1*m5*sin(2*q2 + 2*q3 + 2*q4))/2 - (dc6^2*dq1*m6*sin(2*q2 + 2*q3 + 2*q4 - 2*q5))/8 - (dc6*dq1*l3*m6*cos(q4 - q5))/4 - (d5*dc6*dq1*m6*sin(2*q2 + 2*q3 + 2*q4 - q5))/2 + (dc6*dq1*l2*m6*cos(q3 + q4 + q5))/4 - (dc6*dq1*l2*m6*cos(2*q2 + q3 + q4 - q5))/4 + (dc6*dq1*l3*m6*cos(2*q2 + 2*q3 + q4 + q5))/4 - (d5*dq1*l2*m6*cos(2*q2 + q3 + q4))/2 - (dc5*dq1*l2*m5*cos(2*q2 + q3 + q4))/2 - (dc6*dq1*l2*m6*cos(q3 + q4 - q5))/4 - (d5*dq1*l2*m6*cos(q3 + q4))/2 - (dc5*dq1*l2*m5*cos(q3 + q4))/2 + (dc6*dq1*l3*m6*cos(q4 + q5))/4 - (dc6*dq1*l3*m6*cos(2*q2 + 2*q3 + q4 - q5))/4 + (d5*dc6*dq1*m6*sin(2*q2 + 2*q3 + 2*q4 + q5))/2 - (d5*dq1*l3*m6*cos(q4))/2 - (d5*dq1*l3*m6*cos(2*q2 + 2*q3 + q4))/2 - (dc5*dq1*l3*m5*cos(q4))/2 - (dc5*dq1*l3*m5*cos(2*q2 + 2*q3 + q4))/2 + (dc6*dq1*l2*m6*cos(2*q2 + q3 + q4 + q5))/4;
C(4,2) = - dq2*(l2*cos(q3 + q4) + l3*cos(q4))*(d5*m6 + dc5*m5) - dc6*dq2*l3*m6*sin(q4)*sin(q5) - dc6*dq2*l2*m6*cos(q3)*sin(q4)*sin(q5) - dc6*dq2*l2*m6*cos(q4)*sin(q3)*sin(q5);
C(4,3) = -l3*(2*dq2 + dq3)*(d5*m6*cos(q4) + dc5*m5*cos(q4) + dc6*m6*sin(q4)*sin(q5));
C(4,4) = 0;
C(4,5) = (dc6*m6*(2*d5*dq5*sin(q5) + 2*d5*dq1*sin(q2 + q3 + q4 - q5) + dc6*dq1*sin(q2 + q3 + q4 - 2*q5) + dc6*dq1*sin(q2 + q3 + q4 + 2*q5) - 2*dc6*dq1*sin(q2 + q3 + q4) + 2*dc6*dq2*sin(2*q5) + 2*dc6*dq3*sin(2*q5) + 2*dc6*dq4*sin(2*q5) - 2*d5*dq1*sin(q2 + q3 + q4 + q5)))/2;
C(4,6) = 0;

C(5,1) = (dc6*dq1*m6*(2*dc6*sin(2*q5) + 2*l2*cos(2*q2 + q3 + q4 - q5) + 2*l3*cos(2*q2 + 2*q3 + q4 + q5) + 2*l2*cos(q3 + q4 - q5) + 2*l3*cos(q4 + q5) + 2*l3*cos(2*q2 + 2*q3 + q4 - q5) + 2*d5*sin(2*q2 + 2*q3 + 2*q4 + q5) + 8*d4*sin(q5) + 2*l2*cos(2*q2 + q3 + q4 + q5) + 2*l3*cos(q4 - q5) + 2*d5*sin(2*q2 + 2*q3 + 2*q4 - q5) + dc6*sin(2*q2 + 2*q3 + 2*q4 - 2*q5) - dc6*sin(2*q2 + 2*q3 + 2*q4 + 2*q5) + 2*l2*cos(q3 + q4 + q5)))/8;
C(5,2) = (dc6*m6*(dq2*l3*cos(q4 - q5) - dc6*dq1*sin(q2 + q3 + q4 - 2*q5) - dc6*dq1*sin(q2 + q3 + q4 + 2*q5) - 2*dq1*l2*cos(q2 - q5) - 2*d5*dq1*sin(q2 + q3 + q4 - q5) + 2*dq1*l3*cos(q2 + q3 + q5) + dq2*l2*cos(q3 + q4 + q5) + 2*dc6*dq1*sin(q2 + q3 + q4) - dc6*dq2*sin(2*q5) - 2*dq1*l3*cos(q2 + q3 - q5) + dq2*l2*cos(q3 + q4 - q5) + 2*d5*dq1*sin(q2 + q3 + q4 + q5) + 2*dq1*l2*cos(q2 + q5) + dq2*l3*cos(q4 + q5)))/2;
C(5,3) = (dc6*m6*(2*dq2*l3*cos(q4 - q5) - dc6*dq1*sin(q2 + q3 + q4 - 2*q5) - dc6*dq1*sin(q2 + q3 + q4 + 2*q5) - 2*d5*dq1*sin(q2 + q3 + q4 - q5) + dq3*l3*cos(q4 - q5) + 2*dq1*l3*cos(q2 + q3 + q5) + 2*dc6*dq1*sin(q2 + q3 + q4) - 2*dc6*dq2*sin(2*q5) - dc6*dq3*sin(2*q5) - 2*dq1*l3*cos(q2 + q3 - q5) + 2*d5*dq1*sin(q2 + q3 + q4 + q5) + 2*dq2*l3*cos(q4 + q5) + dq3*l3*cos(q4 + q5)))/2;
C(5,4) = -(dc6*m6*(2*d5*dq1*sin(q2 + q3 + q4 - q5) + dc6*dq1*sin(q2 + q3 + q4 - 2*q5) + dc6*dq1*sin(q2 + q3 + q4 + 2*q5) - 2*dc6*dq1*sin(q2 + q3 + q4) + 2*dc6*dq2*sin(2*q5) + 2*dc6*dq3*sin(2*q5) + dc6*dq4*sin(2*q5) - 2*d5*dq1*sin(q2 + q3 + q4 + q5)))/2;
C(5,5) = 0;
C(5,6) = 0;

C(6,1) = 0;
C(6,2) = 0;
C(6,3) = 0;
C(6,4) = 0;
C(6,5) = 0;
C(6,6) = 0;


% Matriz de Gravedad G: 

G = zeros(6,1);

G(1,1) = 0;

G(2,1) = l2*m3*cos(q2) + l2*m4*cos(q2) + l2*m5*cos(q2) + l2*m6*cos(q2) + lc2*m2*cos(q2) + (dc6*m6*sin(q2 + q3 + q4 - q5))/2 + d5*m6*sin(q2 + q3 + q4) + dc5*m5*sin(q2 + q3 + q4) - (dc6*m6*sin(q2 + q3 + q4 + q5))/2 + l3*m4*cos(q2 + q3) + l3*m5*cos(q2 + q3) + l3*m6*cos(q2 + q3) + lc3*m3*cos(q2 + q3);

G(3,1) = (dc6*m6*sin(q2 + q3 + q4 - q5))/2 + d5*m6*sin(q2 + q3 + q4) + dc5*m5*sin(q2 + q3 + q4) - (dc6*m6*sin(q2 + q3 + q4 + q5))/2 + l3*m4*cos(q2 + q3) + l3*m5*cos(q2 + q3) + l3*m6*cos(q2 + q3) + lc3*m3*cos(q2 + q3);

G(4,1) = (dc6*m6*sin(q2 + q3 + q4 - q5))/2 + d5*m6*sin(q2 + q3 + q4) + dc5*m5*sin(q2 + q3 + q4) - (dc6*m6*sin(q2 + q3 + q4 + q5))/2;

G(5,1) = -(dc6*m6*(sin(q2 + q3 + q4 + q5) + sin(q2 + q3 + q4 - q5)))/2;

G(6,1) = 0;





ddq = D^-1*(-C*dq-G*g+(tau_R-tau_L));

== matlab function modelo_robot_6dof_dindir/q to xyz ==
  data: robot_params input; p output size=[3,6]; q input size=[6,1]; dq input size=[6,1]; ddq input size=[6,1]; dp output size=[3,1]; ddp output size=[3,1]
function [p,dp,ddp] = fcn(robot_params,q,dq,ddq)

%l1 = robot_params.l(1);
l2 = robot_params.l(2);
l3 = robot_params.l(3);
%l4 = robot_params.l(4);
%l5 = robot_params.l(5);
%l6 = robot_params.l(6);

lc1 = robot_params.lc(1);
lc2 = robot_params.lc(2);
lc3 = robot_params.lc(3);
%lc4 = robot_params.lc(4);
%lc5 = robot_params.lc(5);
%lc6 = robot_params.lc(6);

d1 = robot_params.d(1);
%d2 = robot_params.d(2);
%d3 = robot_params.d(3);
d4 = robot_params.d(4);
d5 = robot_params.d(5);
d6 = robot_params.d(6);

dc1 = robot_params.dc(1);
%dc2 = robot_params.dc(2);
%dc3 = robot_params.dc(3);
dc4 = robot_params.dc(4);
dc5 = robot_params.dc(5);
dc6 = robot_params.dc(6);

% %yc1 = 0;%robot_params.yc(1);
% yc2 = 0;%robot_params.yc(2);
% yc3 = 0;%robot_params.yc(3);
% yc4 = 0;%robot_params.yc(4);
% %yc5 = 0;%robot_params.yc(5);
% yc6 = 0;%robot_params.yc(6);

q1 = q(1);
q2 = q(2);
q3 = q(3);
q4 = q(4);
q5 = q(5);
q6 = q(6);


% Cinematica directa %%%%%%%%%%%%%%%%%%%%%%%%%%%%%%%%%%%%%%%%%%%%%%%%%%%%%%

DH = [0   pi/2  d1 q1;
      l2  0     0  q2;
      l3  0     0  q3;
      0   pi/2  d4 q4;
      0   -pi/2 d5 q5;
      0   0     d6 q6];

A01 = transformacion_homogenea(DH(1,:));
A12 = transformacion_homogenea(DH(2,:));
A23 = transformacion_homogenea(DH(3,:));
A34 = transformacion_homogenea(DH(4,:));
A45 = transformacion_homogenea(DH(5,:));
A56 = transformacion_homogenea(DH(6,:));

T0 = zeros(4,4,6);

T0(:,:,1) = A01;
T0(:,:,2) = A01*A12;
T0(:,:,3) = A01*A12*A23;
T0(:,:,4) = A01*A12*A23*A34;
T0(:,:,5) = A01*A12*A23*A34*A45;
T0(:,:,6) = A01*A12*A23*A34*A45*A56;

p = reshape(T0(1:3,4,:),[3,6]);


% Cinematica diferencial %%%%%%%%%%%%%%%%%%%%%%%%%%%%%%%%%%%%%%%%%%%%%%%%%%
JP = zeros(3,6);

JP(1,1) = -cos(q1)*(d1 + l3*sin(q2 + q3) + l2*sin(q2) - d5*cos(q2 + q3 + q4) - dc6*sin(q2 + q3 + q4)*sin(q5));
JP(1,2) = -cos(q1)*(d1 - dc1 + l3*sin(q2 + q3) + l2*sin(q2) - d5*cos(q2 + q3 + q4) - dc6*sin(q2 + q3 + q4)*sin(q5));
JP(1,3) = cos(q1)*(lc2*sin(q2) - l2*sin(q2) - l3*sin(q2 + q3) + d5*cos(q2 + q3 + q4) + dc6*sin(q2 + q3 + q4)*sin(q5));
JP(1,4) = - cos(q2 + q3 + q4)*(dc6*(cos(q1)*cos(q5) + cos(q2 + q3 + q4)*sin(q1)*sin(q5)) + d4*cos(q1) - sin(q1)*(l3*cos(q2 + q3) + l2*cos(q2)) + sin(q1)*(lc3*cos(q2 + q3) + l2*cos(q2)) - d5*sin(q2 + q3 + q4)*sin(q1)) - sin(q2 + q3 + q4)*sin(q1)*(lc3*sin(q2 + q3) - l3*sin(q2 + q3) + d5*cos(q2 + q3 + q4) + dc6*sin(q2 + q3 + q4)*sin(q5));
JP(1,5) = d5*sin(q1)*sin(q5) + d5*cos(q2 + q3 + q4)*cos(q1)*cos(q5) - d4*sin(q2 + q3 + q4)*cos(q1)*sin(q5) + dc4*sin(q2 + q3 + q4)*cos(q1)*sin(q5);
JP(1,6) = (d5 - dc5)*(sin(q1)*sin(q5) + cos(q2 + q3 + q4)*cos(q1)*cos(q5));

JP(2,1) = -sin(q1)*(d1 + l3*sin(q2 + q3) + l2*sin(q2) - d5*cos(q2 + q3 + q4) - dc6*sin(q2 + q3 + q4)*sin(q5));
JP(2,2) = -sin(q1)*(d1 - dc1 + l3*sin(q2 + q3) + l2*sin(q2) - d5*cos(q2 + q3 + q4) - dc6*sin(q2 + q3 + q4)*sin(q5));
JP(2,3) = sin(q1)*(lc2*sin(q2) - l2*sin(q2) - l3*sin(q2 + q3) + d5*cos(q2 + q3 + q4) + dc6*sin(q2 + q3 + q4)*sin(q5));
JP(2,4) = sin(q2 + q3 + q4)*cos(q1)*(lc3*sin(q2 + q3) - l3*sin(q2 + q3) + d5*cos(q2 + q3 + q4) + dc6*sin(q2 + q3 + q4)*sin(q5)) - cos(q2 + q3 + q4)*(dc6*(cos(q5)*sin(q1) - cos(q2 + q3 + q4)*cos(q1)*sin(q5)) + cos(q1)*(l3*cos(q2 + q3) + l2*cos(q2)) - cos(q1)*(lc3*cos(q2 + q3) + l2*cos(q2)) + d4*sin(q1) + d5*sin(q2 + q3 + q4)*cos(q1));
JP(2,5) = d5*cos(q2 + q3 + q4)*cos(q5)*sin(q1) - d5*cos(q1)*sin(q5) - d4*sin(q2 + q3 + q4)*sin(q1)*sin(q5) + dc4*sin(q2 + q3 + q4)*sin(q1)*sin(q5);
JP(2,6) = -(d5 - dc5)*(cos(q1)*sin(q5) - cos(q2 + q3 + q4)*cos(q5)*sin(q1));

JP(3,1) = l3*cos(q2 + q3) - (dc6*sin(q2 + q3 + q4 + q5))/2 + l2*cos(q2) + (dc6*sin(q2 + q3 + q4 - q5))/2 + d5*sin(q2 + q3 + q4);
JP(3,2) = l3*cos(q2 + q3) - (dc6*sin(q2 + q3 + q4 + q5))/2 - lc1 + l2*cos(q2) + (dc6*sin(q2 + q3 + q4 - q5))/2 + d5*sin(q2 + q3 + q4);
JP(3,3) = l3*cos(q2 + q3) - (dc6*sin(q2 + q3 + q4 + q5))/2 + l2*cos(q2) - lc2*cos(q2) + (dc6*sin(q2 + q3 + q4 - q5))/2 + d5*sin(q2 + q3 + q4);
JP(3,4) = - (dc6*sin(q2 + q3 + q4 + q5))/2 - (dc6*sin(q2 + q3 + q4 - q5))/2 - d4*sin(q2 + q3 + q4);
JP(3,5) = d4*cos(q2 + q3 + q4)*sin(q5) + d5*sin(q2 + q3 + q4)*cos(q5) - dc4*cos(q2 + q3 + q4)*sin(q5);
JP(3,6) = sin(q2 + q3 + q4)*cos(q5)*(d5 - dc5);

dp = JP*dq;

dq1 = dq(1);
dq2 = dq(2);
dq3 = dq(3);
dq4 = dq(4);
dq5 = dq(5);
%dq6 = dq(6);

dJP = zeros(3,6);

dJP(1,1) = dq1*sin(q1)*(d1 + l3*sin(q2 + q3) + l2*sin(q2) - d5*cos(q2 + q3 + q4) - dc6*sin(q2 + q3 + q4)*sin(q5)) - dq3*cos(q1)*(l3*cos(q2 + q3) + d5*sin(q2 + q3 + q4) - dc6*cos(q2 + q3 + q4)*sin(q5)) - dq4*cos(q1)*(d5*sin(q2 + q3 + q4) - dc6*cos(q2 + q3 + q4)*sin(q5)) - dq2*cos(q1)*(l3*cos(q2 + q3) + l2*cos(q2) + d5*sin(q2 + q3 + q4) - dc6*cos(q2 + q3 + q4)*sin(q5)) + dc6*dq5*sin(q2 + q3 + q4)*cos(q1)*cos(q5);
dJP(1,2) = dq1*sin(q1)*(d1 - dc1 + l3*sin(q2 + q3) + l2*sin(q2) - d5*cos(q2 + q3 + q4) - dc6*sin(q2 + q3 + q4)*sin(q5)) - dq3*cos(q1)*(l3*cos(q2 + q3) + d5*sin(q2 + q3 + q4) - dc6*cos(q2 + q3 + q4)*sin(q5)) - dq4*cos(q1)*(d5*sin(q2 + q3 + q4) - dc6*cos(q2 + q3 + q4)*sin(q5)) - dq2*cos(q1)*(l3*cos(q2 + q3) + l2*cos(q2) + d5*sin(q2 + q3 + q4) - dc6*cos(q2 + q3 + q4)*sin(q5)) + dc6*dq5*sin(q2 + q3 + q4)*cos(q1)*cos(q5);
dJP(1,3) = dc6*dq5*sin(q2 + q3 + q4)*cos(q1)*cos(q5) - dq2*cos(q1)*(l3*cos(q2 + q3) + l2*cos(q2) - lc2*cos(q2) + d5*sin(q2 + q3 + q4) - dc6*cos(q2 + q3 + q4)*sin(q5)) - dq1*sin(q1)*(lc2*sin(q2) - l2*sin(q2) - l3*sin(q2 + q3) + d5*cos(q2 + q3 + q4) + dc6*sin(q2 + q3 + q4)*sin(q5)) - dq4*cos(q1)*(d5*sin(q2 + q3 + q4) - dc6*cos(q2 + q3 + q4)*sin(q5)) - dq3*cos(q1)*(l3*cos(q2 + q3) + d5*sin(q2 + q3 + q4) - dc6*cos(q2 + q3 + q4)*sin(q5));
dJP(1,4) = dq1*l3*cos(q1)*cos(q4) - dq1*lc3*cos(q1)*cos(q4) - dc6*dq1*cos(q1)*sin(q5) - dc6*dq5*cos(q5)*sin(q1) - dq4*l3*sin(q1)*sin(q4) + dq4*lc3*sin(q1)*sin(q4) + d4*dq1*cos(q2)*cos(q3)*cos(q4)*sin(q1) + d4*dq2*cos(q1)*cos(q2)*cos(q3)*sin(q4) + d4*dq2*cos(q1)*cos(q2)*cos(q4)*sin(q3) + d4*dq2*cos(q1)*cos(q3)*cos(q4)*sin(q2) + d4*dq3*cos(q1)*cos(q2)*cos(q3)*sin(q4) + d4*dq3*cos(q1)*cos(q2)*cos(q4)*sin(q3) + d4*dq3*cos(q1)*cos(q3)*cos(q4)*sin(q2) + d4*dq4*cos(q1)*cos(q2)*cos(q3)*sin(q4) + d4*dq4*cos(q1)*cos(q2)*cos(q4)*sin(q3) + d4*dq4*cos(q1)*cos(q3)*cos(q4)*sin(q2) - d4*dq1*cos(q2)*sin(q1)*sin(q3)*sin(q4) - d4*dq1*cos(q3)*sin(q1)*sin(q2)*sin(q4) - d4*dq1*cos(q4)*sin(q1)*sin(q2)*sin(q3) - d4*dq2*cos(q1)*sin(q2)*sin(q3)*sin(q4) - d4*dq3*cos(q1)*sin(q2)*sin(q3)*sin(q4) - d4*dq4*cos(q1)*sin(q2)*sin(q3)*sin(q4) + dc6*dq1*cos(q2)*cos(q3)*cos(q4)*cos(q5)*sin(q1) + dc6*dq2*cos(q1)*cos(q2)*cos(q3)*cos(q5)*sin(q4) + dc6*dq2*cos(q1)*cos(q2)*cos(q4)*cos(q5)*sin(q3) + dc6*dq2*cos(q1)*cos(q3)*cos(q4)*cos(q5)*sin(q2) + dc6*dq3*cos(q1)*cos(q2)*cos(q3)*cos(q5)*sin(q4) + dc6*dq3*cos(q1)*cos(q2)*cos(q4)*cos(q5)*sin(q3) + dc6*dq3*cos(q1)*cos(q3)*cos(q4)*cos(q5)*sin(q2) + dc6*dq4*cos(q1)*cos(q2)*cos(q3)*cos(q5)*sin(q4) + dc6*dq4*cos(q1)*cos(q2)*cos(q4)*cos(q5)*sin(q3) + dc6*dq4*cos(q1)*cos(q3)*cos(q4)*cos(q5)*sin(q2) + dc6*dq5*cos(q1)*cos(q2)*cos(q3)*cos(q4)*sin(q5) - dc6*dq1*cos(q2)*cos(q5)*sin(q1)*sin(q3)*sin(q4) - dc6*dq1*cos(q3)*cos(q5)*sin(q1)*sin(q2)*sin(q4) - dc6*dq1*cos(q4)*cos(q5)*sin(q1)*sin(q2)*sin(q3) - dc6*dq2*cos(q1)*cos(q5)*sin(q2)*sin(q3)*sin(q4) - dc6*dq3*cos(q1)*cos(q5)*sin(q2)*sin(q3)*sin(q4) - dc6*dq4*cos(q1)*cos(q5)*sin(q2)*sin(q3)*sin(q4) - dc6*dq5*cos(q1)*cos(q2)*sin(q3)*sin(q4)*sin(q5) - dc6*dq5*cos(q1)*cos(q3)*sin(q2)*sin(q4)*sin(q5) - dc6*dq5*cos(q1)*cos(q4)*sin(q2)*sin(q3)*sin(q5);
dJP(1,5) = dq5*(d5*cos(q5)*sin(q1) - d4*sin(q2 + q3 + q4)*cos(q1)*cos(q5) - d5*cos(q2 + q3 + q4)*cos(q1)*sin(q5) + dc4*sin(q2 + q3 + q4)*cos(q1)*cos(q5)) + dq1*(d5*cos(q1)*sin(q5) - d5*cos(q2 + q3 + q4)*cos(q5)*sin(q1) + d4*sin(q2 + q3 + q4)*sin(q1)*sin(q5) - dc4*sin(q2 + q3 + q4)*sin(q1)*sin(q5)) - dq2*cos(q1)*(d4*cos(q2 + q3 + q4)*sin(q5) + d5*sin(q2 + q3 + q4)*cos(q5) - dc4*cos(q2 + q3 + q4)*sin(q5)) - dq3*cos(q1)*(d4*cos(q2 + q3 + q4)*sin(q5) + d5*sin(q2 + q3 + q4)*cos(q5) - dc4*cos(q2 + q3 + q4)*sin(q5)) - dq4*cos(q1)*(d4*cos(q2 + q3 + q4)*sin(q5) + d5*sin(q2 + q3 + q4)*cos(q5) - dc4*cos(q2 + q3 + q4)*sin(q5));
dJP(1,6) = dq1*(d5 - dc5)*(cos(q1)*sin(q5) - cos(q2 + q3 + q4)*cos(q5)*sin(q1)) + dq5*(d5 - dc5)*(cos(q5)*sin(q1) - cos(q2 + q3 + q4)*cos(q1)*sin(q5)) - dq2*sin(q2 + q3 + q4)*cos(q1)*cos(q5)*(d5 - dc5) - dq3*sin(q2 + q3 + q4)*cos(q1)*cos(q5)*(d5 - dc5) - dq4*sin(q2 + q3 + q4)*cos(q1)*cos(q5)*(d5 - dc5);

dJP(2,1) = dc6*dq5*sin(q2 + q3 + q4)*cos(q5)*sin(q1) - dq1*cos(q1)*(d1 + l3*sin(q2 + q3) + l2*sin(q2) - d5*cos(q2 + q3 + q4) - dc6*sin(q2 + q3 + q4)*sin(q5)) - dq4*sin(q1)*(d5*sin(q2 + q3 + q4) - dc6*cos(q2 + q3 + q4)*sin(q5)) - dq2*sin(q1)*(l3*cos(q2 + q3) + l2*cos(q2) + d5*sin(q2 + q3 + q4) - dc6*cos(q2 + q3 + q4)*sin(q5)) - dq3*sin(q1)*(l3*cos(q2 + q3) + d5*sin(q2 + q3 + q4) - dc6*cos(q2 + q3 + q4)*sin(q5));
dJP(2,2) = dc6*dq5*sin(q2 + q3 + q4)*cos(q5)*sin(q1) - dq4*sin(q1)*(d5*sin(q2 + q3 + q4) - dc6*cos(q2 + q3 + q4)*sin(q5)) - dq2*sin(q1)*(l3*cos(q2 + q3) + l2*cos(q2) + d5*sin(q2 + q3 + q4) - dc6*cos(q2 + q3 + q4)*sin(q5)) - dq1*cos(q1)*(d1 - dc1 + l3*sin(q2 + q3) + l2*sin(q2) - d5*cos(q2 + q3 + q4) - dc6*sin(q2 + q3 + q4)*sin(q5)) - dq3*sin(q1)*(l3*cos(q2 + q3) + d5*sin(q2 + q3 + q4) - dc6*cos(q2 + q3 + q4)*sin(q5));
dJP(2,3) = dq1*cos(q1)*(lc2*sin(q2) - l2*sin(q2) - l3*sin(q2 + q3) + d5*cos(q2 + q3 + q4) + dc6*sin(q2 + q3 + q4)*sin(q5)) - dq2*sin(q1)*(l3*cos(q2 + q3) + l2*cos(q2) - lc2*cos(q2) + d5*sin(q2 + q3 + q4) - dc6*cos(q2 + q3 + q4)*sin(q5)) - dq3*sin(q1)*(l3*cos(q2 + q3) + d5*sin(q2 + q3 + q4) - dc6*cos(q2 + q3 + q4)*sin(q5)) - dq4*sin(q1)*(d5*sin(q2 + q3 + q4) - dc6*cos(q2 + q3 + q4)*sin(q5)) + dc6*dq5*sin(q2 + q3 + q4)*cos(q5)*sin(q1);
dJP(2,4) = dc6*dq5*cos(q1)*cos(q5) + dq1*l3*cos(q4)*sin(q1) + dq4*l3*cos(q1)*sin(q4) - dq1*lc3*cos(q4)*sin(q1) - dq4*lc3*cos(q1)*sin(q4) - dc6*dq1*sin(q1)*sin(q5) - d4*dq1*cos(q1)*cos(q2)*cos(q3)*cos(q4) + d4*dq1*cos(q1)*cos(q2)*sin(q3)*sin(q4) + d4*dq1*cos(q1)*cos(q3)*sin(q2)*sin(q4) + d4*dq1*cos(q1)*cos(q4)*sin(q2)*sin(q3) + d4*dq2*cos(q2)*cos(q3)*sin(q1)*sin(q4) + d4*dq2*cos(q2)*cos(q4)*sin(q1)*sin(q3) + d4*dq2*cos(q3)*cos(q4)*sin(q1)*sin(q2) + d4*dq3*cos(q2)*cos(q3)*sin(q1)*sin(q4) + d4*dq3*cos(q2)*cos(q4)*sin(q1)*sin(q3) + d4*dq3*cos(q3)*cos(q4)*sin(q1)*sin(q2) + d4*dq4*cos(q2)*cos(q3)*sin(q1)*sin(q4) + d4*dq4*cos(q2)*cos(q4)*sin(q1)*sin(q3) + d4*dq4*cos(q3)*cos(q4)*sin(q1)*sin(q2) - d4*dq2*sin(q1)*sin(q2)*sin(q3)*sin(q4) - d4*dq3*sin(q1)*sin(q2)*sin(q3)*sin(q4) - d4*dq4*sin(q1)*sin(q2)*sin(q3)*sin(q4) - dc6*dq1*cos(q1)*cos(q2)*cos(q3)*cos(q4)*cos(q5) + dc6*dq1*cos(q1)*cos(q2)*cos(q5)*sin(q3)*sin(q4) + dc6*dq1*cos(q1)*cos(q3)*cos(q5)*sin(q2)*sin(q4) + dc6*dq1*cos(q1)*cos(q4)*cos(q5)*sin(q2)*sin(q3) + dc6*dq2*cos(q2)*cos(q3)*cos(q5)*sin(q1)*sin(q4) + dc6*dq2*cos(q2)*cos(q4)*cos(q5)*sin(q1)*sin(q3) + dc6*dq2*cos(q3)*cos(q4)*cos(q5)*sin(q1)*sin(q2) + dc6*dq3*cos(q2)*cos(q3)*cos(q5)*sin(q1)*sin(q4) + dc6*dq3*cos(q2)*cos(q4)*cos(q5)*sin(q1)*sin(q3) + dc6*dq3*cos(q3)*cos(q4)*cos(q5)*sin(q1)*sin(q2) + dc6*dq4*cos(q2)*cos(q3)*cos(q5)*sin(q1)*sin(q4) + dc6*dq4*cos(q2)*cos(q4)*cos(q5)*sin(q1)*sin(q3) + dc6*dq4*cos(q3)*cos(q4)*cos(q5)*sin(q1)*sin(q2) + dc6*dq5*cos(q2)*cos(q3)*cos(q4)*sin(q1)*sin(q5) - dc6*dq2*cos(q5)*sin(q1)*sin(q2)*sin(q3)*sin(q4) - dc6*dq3*cos(q5)*sin(q1)*sin(q2)*sin(q3)*sin(q4) - dc6*dq4*cos(q5)*sin(q1)*sin(q2)*sin(q3)*sin(q4) - dc6*dq5*cos(q2)*sin(q1)*sin(q3)*sin(q4)*sin(q5) - dc6*dq5*cos(q3)*sin(q1)*sin(q2)*sin(q4)*sin(q5) - dc6*dq5*cos(q4)*sin(q1)*sin(q2)*sin(q3)*sin(q5);
dJP(2,5) = dq1*(d5*sin(q1)*sin(q5) + d5*cos(q2 + q3 + q4)*cos(q1)*cos(q5) - d4*sin(q2 + q3 + q4)*cos(q1)*sin(q5) + dc4*sin(q2 + q3 + q4)*cos(q1)*sin(q5)) - dq5*(d5*cos(q1)*cos(q5) + d4*sin(q2 + q3 + q4)*cos(q5)*sin(q1) + d5*cos(q2 + q3 + q4)*sin(q1)*sin(q5) - dc4*sin(q2 + q3 + q4)*cos(q5)*sin(q1)) - dq2*sin(q1)*(d4*cos(q2 + q3 + q4)*sin(q5) + d5*sin(q2 + q3 + q4)*cos(q5) - dc4*cos(q2 + q3 + q4)*sin(q5)) - dq3*sin(q1)*(d4*cos(q2 + q3 + q4)*sin(q5) + d5*sin(q2 + q3 + q4)*cos(q5) - dc4*cos(q2 + q3 + q4)*sin(q5)) - dq4*sin(q1)*(d4*cos(q2 + q3 + q4)*sin(q5) + d5*sin(q2 + q3 + q4)*cos(q5) - dc4*cos(q2 + q3 + q4)*sin(q5));
dJP(2,6) = dq1*(d5 - dc5)*(sin(q1)*sin(q5) + cos(q2 + q3 + q4)*cos(q1)*cos(q5)) - dq5*(d5 - dc5)*(cos(q1)*cos(q5) + cos(q2 + q3 + q4)*sin(q1)*sin(q5)) - dq2*sin(q2 + q3 + q4)*cos(q5)*sin(q1)*(d5 - dc5) - dq3*sin(q2 + q3 + q4)*cos(q5)*sin(q1)*(d5 - dc5) - dq4*sin(q2 + q3 + q4)*cos(q5)*sin(q1)*(d5 - dc5);

dJP(3,1) = dq4*((dc6*cos(q2 + q3 + q4 - q5))/2 - (dc6*cos(q2 + q3 + q4 + q5))/2 + d5*cos(q2 + q3 + q4)) - dq3*((dc6*cos(q2 + q3 + q4 + q5))/2 + l3*sin(q2 + q3) - (dc6*cos(q2 + q3 + q4 - q5))/2 - d5*cos(q2 + q3 + q4)) - dq2*((dc6*cos(q2 + q3 + q4 + q5))/2 + l3*sin(q2 + q3) - (dc6*cos(q2 + q3 + q4 - q5))/2 + l2*sin(q2) - d5*cos(q2 + q3 + q4)) - (dc6*dq5*(cos(q2 + q3 + q4 + q5) + cos(q2 + q3 + q4 - q5)))/2;
dJP(3,2) = dq4*((dc6*cos(q2 + q3 + q4 - q5))/2 - (dc6*cos(q2 + q3 + q4 + q5))/2 + d5*cos(q2 + q3 + q4)) - dq3*((dc6*cos(q2 + q3 + q4 + q5))/2 + l3*sin(q2 + q3) - (dc6*cos(q2 + q3 + q4 - q5))/2 - d5*cos(q2 + q3 + q4)) - dq2*((dc6*cos(q2 + q3 + q4 + q5))/2 + l3*sin(q2 + q3) - (dc6*cos(q2 + q3 + q4 - q5))/2 + l2*sin(q2) - d5*cos(q2 + q3 + q4)) - (dc6*dq5*(cos(q2 + q3 + q4 + q5) + cos(q2 + q3 + q4 - q5)))/2;
dJP(3,3) = dq4*((dc6*cos(q2 + q3 + q4 - q5))/2 - (dc6*cos(q2 + q3 + q4 + q5))/2 + d5*cos(q2 + q3 + q4)) - dq3*((dc6*cos(q2 + q3 + q4 + q5))/2 + l3*sin(q2 + q3) - (dc6*cos(q2 + q3 + q4 - q5))/2 - d5*cos(q2 + q3 + q4)) - dq2*((dc6*cos(q2 + q3 + q4 + q5))/2 + l3*sin(q2 + q3) - (dc6*cos(q2 + q3 + q4 - q5))/2 + l2*sin(q2) - lc2*sin(q2) - d5*cos(q2 + q3 + q4)) - dq5*((dc6*cos(q2 + q3 + q4 + q5))/2 + (dc6*cos(q2 + q3 + q4 - q5))/2);
dJP(3,4) = - dq2*((dc6*cos(q2 + q3 + q4 + q5))/2 + (dc6*cos(q2 + q3 + q4 - q5))/2 + d4*cos(q2 + q3 + q4)) - dq3*((dc6*cos(q2 + q3 + q4 + q5))/2 + (dc6*cos(q2 + q3 + q4 - q5))/2 + d4*cos(q2 + q3 + q4)) - dq4*((dc6*cos(q2 + q3 + q4 + q5))/2 + (dc6*cos(q2 + q3 + q4 - q5))/2 + d4*cos(q2 + q3 + q4)) - (dc6*dq5*(cos(q2 + q3 + q4 + q5) - cos(q2 + q3 + q4 - q5)))/2;
dJP(3,5) = dq2*(d5*cos(q2 + q3 + q4)*cos(q5) - d4*sin(q2 + q3 + q4)*sin(q5) + dc4*sin(q2 + q3 + q4)*sin(q5)) - dq5*(dc4*cos(q2 + q3 + q4)*cos(q5) - d4*cos(q2 + q3 + q4)*cos(q5) + d5*sin(q2 + q3 + q4)*sin(q5)) + dq3*(d5*cos(q2 + q3 + q4)*cos(q5) - d4*sin(q2 + q3 + q4)*sin(q5) + dc4*sin(q2 + q3 + q4)*sin(q5)) + dq4*(d5*cos(q2 + q3 + q4)*cos(q5) - d4*sin(q2 + q3 + q4)*sin(q5) + dc4*sin(q2 + q3 + q4)*sin(q5));
dJP(3,6) = (d5 - dc5)*(dq2*cos(q2 + q3 + q4)*cos(q5) + dq3*cos(q2 + q3 + q4)*cos(q5) + dq4*cos(q2 + q3 + q4)*cos(q5) - dq5*sin(q2 + q3 + q4)*sin(q5));

ddp = dJP*ddq;

end

function m = transformacion_homogenea(DH_i)
    a_i = DH_i(1);
    alpha_i = DH_i(2);
    d_i = DH_i(3);
    theta_i = DH_i(4);
    
    ma_i = [1 0 0 a_i;
            0 1 0 0;
            0 0 1 0;
            0 0 0 1];
    
    md_i = [1 0 0 0;
            0 1 0 0;
            0 0 1 d_i;
            0 0 0 1];
    
    mtheta_i = [cos(theta_i) -sin(theta_i) 0 0;
                sin(theta_i) cos(theta_i) 0 0;
                0 0 1 0;
                0 0 0 1];
    
    malpha_i = [1 0 0 0;
                0 cos(alpha_i) -sin(alpha_i) 0;
                0 sin(alpha_i) cos(alpha_i) 0;
                0 0 0 1];
    
    m = mtheta_i * md_i * ma_i * malpha_i;

end
